simulink model "Prob_6"  (R2020b)
settings: Solver=VariableStepAuto  StartTime=0.0  StopTime=10  RelTol=1e-3
settings Model: Creator=Akshay A H  LastModifiedBy=Akshay A H

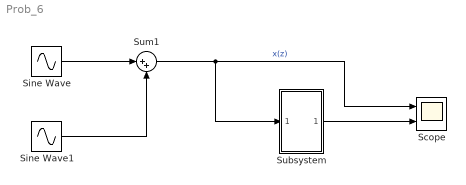
== system Prob_6 ==
  Scope : Scope  NumInputPorts=2
  Sine Wave : Sin  SampleTime=0
  Sine Wave1 : Sin  Amplitude=0.0005  Frequency=2000  SampleTime=0
  Subsystem : ModelReference  ModelNameDialog=Subsystem  SimulationMode=Normal  ModelReferenceVersion=1.4
  Sum1 : Sum  Inputs=|++
  wires:
  Sine Wave/1 -> Sum1/1
  Sine Wave1/1 -> Sum1/2
  Sum1/1 -> Subsystem/1, Scope/1  "x(z)"
  Subsystem/1 -> Scope/2
